simulink model "MPPT"  (R2024b)
settings: Solver=ode1  StartTime=0.0  StopTime=10  FixedStep=5e-6  RelTol=1e-3
libraries: spsSeriesRLCBranchLib x6, spsCurrentMeasurementLib x4, spsVoltageMeasurementLib x3, spsSawtoothGeneratorLib x2, spsBreakerLib x1, spsDiodeLib x1, spsGroundLib x1, spsIGBTDiodeLib x1, spsPVArrayLib x1, sps_lib x1
settings Model: Creator=DSPACE  LastModifiedBy=Ashwin Soni
settings SolverCC: AlgebraicLoopSolver=TrustRegion
settings DebuggingCC: UnconnectedInputMsg=warning  UnconnectedOutputMsg=warning  UnconnectedLineMsg=warning
settings ModelReferenceCC: EnableRefExpFcnMdlSchedulingChecks=on
settings RTWCC: GPUComputeCapability=3.5  DLArmComputeVersion=19.05

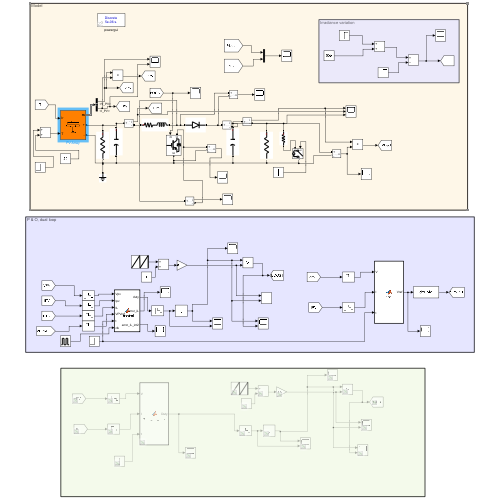
[thumbnail: Simulink's stored preview of the top-level diagram]
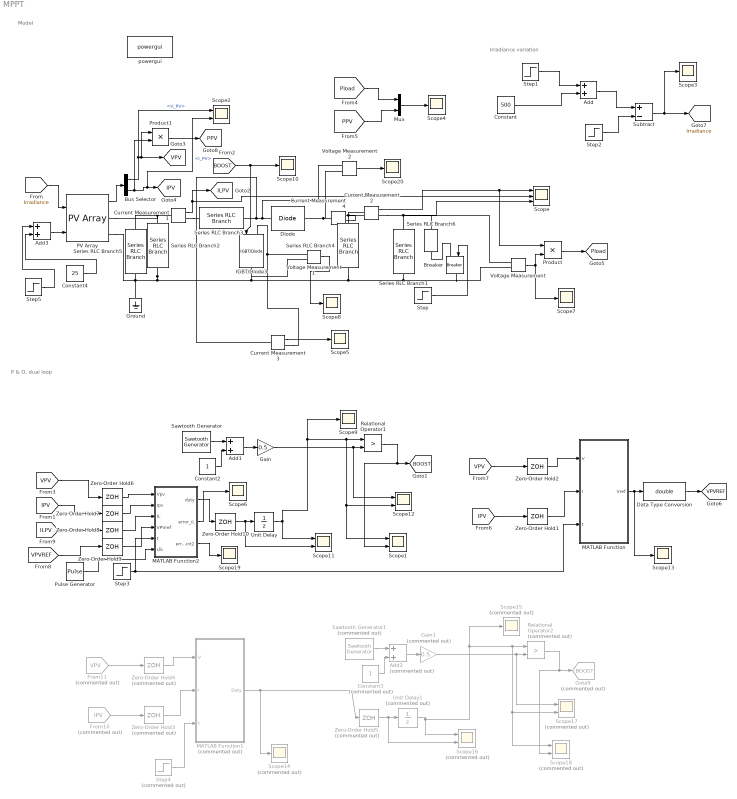
== system MPPT ==
  note: Irradiance variation
  note: Model
  note: P & O, dual loop
  Add : Sum
  Add1 : Sum
  Add2 : Sum  Commented=on
  Add3 : Sum
  Breaker : spsBreakerLib/Breaker  InitialState=0  SwitchingTimes="[1/60  5/60]"  External=on  BreakerResistance=0.01  SnubberResistance=1e6  SnubberCapacitance=inf  Measurements=None  MoreParameters=on  NoBreakLoop=off
  Bus Selector : BusSelector  OutputSignals=V_PV,I_PV
  Constant : Constant  Value=500
  Constant2 : Constant
  Constant3 : Constant  Commented=on
  Constant4 : Constant  Value=25
  Current Measurement{1..4} (4 alike) : spsCurrentMeasurementLib/Current Measurement  PhasorSimulation=off  OutputType=Complex  PSBequivalent=0
  Data Type Conversion : DataTypeConversion  OutDataTypeStr=double  SaturateOnIntegerOverflow=off  RndMeth=Floor
  Diode : spsDiodeLib/Diode  Ron=0.001  Lon=0  Vf=0.8  IC=0  UseSnubber=0  Rs=inf  Cs=250e-9  Measurements=off
  From10 : From  Commented=on  GotoTag=IPV  TagVisibility=global
  From11 : From  Commented=on  GotoTag=VPV  TagVisibility=global
  Gain : Gain  Gain=0.5
  Gain1 : Gain  Commented=on  Gain=0.5
  Goto9 : Goto  Commented=on  GotoTag=BOOST  TagVisibility=global
  Ground : spsGroundLib/Ground  LConnTagsString=a
  IGBT/Diode3 : spsIGBTDiodeLib/IGBT//Diode  Ron=75e-3  Rs=5  Cs=15e-9  Measurements=off
  MATLAB Function : MATLAB Function  TreatAsAtomicUnit=on
  MATLAB Function1 : MATLAB Function  Commented=on  TreatAsAtomicUnit=on
  MATLAB Function2 : MATLAB Function  TreatAsAtomicUnit=on
  Mux : Mux  Inputs=2
  PV Array : spsPVArrayLib/PV Array  Npar=2  Nser=2  PlotType=array @ 25 deg.C & specified irradiances  S_vec="[ 1000  800  600 ]"  Temp_C_vec="[ 45 25  ]"  ModuleName=Advance Solar Hydro Wind Power API-150  PlotWhenSelected=off  Pm=150.075  Ncell=72  Voc=41.8  Isc=5.05  Vm=34.5  Im=4.35  beta_Voc_pc=-0.419  alpha_Isc_pc=0.096  beta_Voc=-0.17514  alpha_Isc=0.004848  IL=5.0762  I0=1.155e-09  nI=1.0233  Rsh=71.9537  Rs=0.37337  RobustModel=off  RobustCellTemperature=313.3991  BAL=on  Tc=1e-6  Tfilter=5e-5
  Product : Product
  Product1 : Product
  Pulse Generator : DiscretePulseGenerator  PulseType=Time based  Period=1e-4  PulseWidth=5
  Relational Operator1 : RelationalOperator  Operator=>  OutDataTypeStr=boolean  RndMeth=Simplest  InputSameDT=off
  Relational Operator2 : RelationalOperator  Commented=on  Operator=>  OutDataTypeStr=boolean  RndMeth=Simplest  InputSameDT=off
  Sawtooth Generator : spsSawtoothGeneratorLib/Sawtooth Generator  Freq=10e3  Phase=0  Ts=0
  Sawtooth Generator1 : spsSawtoothGeneratorLib/Sawtooth Generator  Commented=on  Freq=10e3  Phase=0  Ts=0
  Scope : Scope  NumInputPorts=3
  Scope{1..2,11..12} (4 alike) : Scope  NumInputPorts=2
  Scope{3..10,13,19..20} (11 alike) : Scope
  Scope14 : Scope  Commented=on
  Scope15 : Scope  Commented=on
  Scope16 : Scope  Commented=on  NumInputPorts=2
  Scope17 : Scope  Commented=on  NumInputPorts=2
  Scope18 : Scope  Commented=on  NumInputPorts=2
  Series RLC Branch1 : spsSeriesRLCBranchLib/Series RLC Branch  LConnTagsString=__new0  RConnTagsString=__new0  BranchType=R  Resistance=100  Inductance=10e-3  SetiL0=off  InitialCurrent=0  Capacitance=1e-6  Setx0=off  InitialVoltage=0  Measurements=Branch voltage and current
  Series RLC Branch2 : spsSeriesRLCBranchLib/Series RLC Branch  LConnTagsString=__new0  RConnTagsString=__new0  BranchType=C  Resistance=1  Inductance=1e-3  SetiL0=off  InitialCurrent=0  Capacitance=220e-6  Setx0=off  InitialVoltage=0  Measurements=None
  Series RLC Branch3 : spsSeriesRLCBranchLib/Series RLC Branch  LConnTagsString=__new0  RConnTagsString=__new0  BranchType=RL  Resistance=0.05  Inductance=13.3e-3  SetiL0=off  InitialCurrent=0  Capacitance=1e-6  Setx0=off  InitialVoltage=0  Measurements=None
  Series RLC Branch4 : spsSeriesRLCBranchLib/Series RLC Branch  LConnTagsString=__new0  RConnTagsString=__new0  BranchType=C  Resistance=1  Inductance=1e-3  SetiL0=off  InitialCurrent=0  Capacitance=220e-6  Setx0=off  InitialVoltage=0  Measurements=None
  Series RLC Branch5 : spsSeriesRLCBranchLib/Series RLC Branch  LConnTagsString=__new0  RConnTagsString=__new0  BranchType=R  Resistance=10E6  Inductance=10e-3  SetiL0=off  InitialCurrent=0  Capacitance=1e-6  Setx0=off  InitialVoltage=0  Measurements=None
  Series RLC Branch6 : spsSeriesRLCBranchLib/Series RLC Branch  LConnTagsString=__new0  RConnTagsString=__new0  BranchType=R  Resistance=1000  Inductance=10e-3  SetiL0=off  InitialCurrent=0  Capacitance=1e-6  Setx0=off  InitialVoltage=0  Measurements=None
  Step : Step  Time=4  SampleTime=0
  Step1 : Step  Time=2  After=500  SampleTime=0
  Step2 : Step  Time=4  After=200  SampleTime=0
  Step3 : Step  Time=2  After=5  SampleTime=0
  Step4 : Step  Commented=on  Time=2  After=5  SampleTime=0
  Step5 : Step  Time=7  After=10  SampleTime=0
  Subtract : Sum  Inputs=+-
  Unit Delay : UnitDelay  SampleTime=1e-4  HasFrameUpgradeWarning=on
  Unit Delay1 : UnitDelay  Commented=on  SampleTime=1e-4  HasFrameUpgradeWarning=on
  Voltage Measurement : spsVoltageMeasurementLib/Voltage Measurement  PhasorSimulation=off  OutputType=Complex  PSBequivalent=0
  Voltage Measurement1 : spsVoltageMeasurementLib/Voltage Measurement  PhasorSimulation=off  OutputType=Complex  PSBequivalent=0
  Voltage Measurement2 : spsVoltageMeasurementLib/Voltage Measurement  PhasorSimulation=off  OutputType=Complex  PSBequivalent=0
  Zero-Order Hold1 : ZeroOrderHold  SampleTime=1e-2
  Zero-Order Hold{6..10} (5 alike) : ZeroOrderHold  SampleTime=1e-4
  Zero-Order Hold2 : ZeroOrderHold  SampleTime=1e-2
  Zero-Order Hold3 : ZeroOrderHold  Commented=on  SampleTime=1e-4
  Zero-Order Hold4 : ZeroOrderHold  Commented=on  SampleTime=1e-4
  Zero-Order Hold5 : ZeroOrderHold  Commented=on  SampleTime=1e-4
  powergui : sps_lib/powergui  Priority=1  SimulationMode=Discrete  SampleTime=5e-6  frequency=60  Iterations=50  frequencyindice=0  Pbase=100e6  ErrMax=1e-4  UnitsV=kV  UnitsW=MW  buscounter=0  FunctionMessages=off  echomessages=off  EnableUseOfTLC=off  CurrentSourceSwitches=off  DisableSnubberDevices=off  DisableRonSwitches=off  DisableVfSwitches=off  DisplayEquations=off  AutomaticDiscreteSolvers=off  SolverType=Tustin/Backward Euler (TBE)  Interpol=off  ExternalGateDelay=off  methode=off  Ts=100  x0status=blocks  SPID=on  SwTol=0  HookPort=off  NonlinearTolerance=1e-4  nMaxIteration=100  ContinueOnMaxIteration=off  RestoreLinks=warning  ResistiveCurrentMeasurement=off  Frange=[0:2:500]  Ylog=off  Xlog=on  ShowGrid=off  save=off  variable=ZData  structure=0  ZoomFFT=off  StartTime=0.0  cycles=1  DisplayStyle=1  fundamental=60  FreqAxis=off  MaxFrequency=1000  frequencyindicesteady=1  RmsSteady=1  display=off
  tag scope: BOOST=global, ILPV=global, IPV=global, Irradiance=global, PPV=global, Pload=global, VPV=global, VPVREF=global
  wires:
  Bus Selector/2 -> Product1/2, Scope2/2, [IPV]  "<I_PV>"
  Current Measurement1/1 -> Scope/2, [ILPV]
  PV Array/1 -> Bus Selector/1
  Bus Selector/1 -> Scope2/1, Product1/1, [VPV]  "<V_PV>"
  Current Measurement2/1 -> Product/1, Scope/1
  Gain/1 -> Scope12/1, Relational Operator1/2
  [Pload] -> Mux/1
  [VPV] -> Zero-Order Hold2/1
  [IPV] -> Zero-Order Hold1/1
  Data Type Conversion/1 -> [VPVREF]
  [IPV] -> Zero-Order Hold7/1
  [VPV] -> Zero-Order Hold6/1
  [VPVREF] -> Zero-Order Hold9/1
  [ILPV] -> Zero-Order Hold8/1
  Zero-Order Hold2/1 -> MATLAB Function/1(V)
  Zero-Order Hold1/1 -> MATLAB Function/2(I)
  [Irradiance] -> PV Array/1
  Mux/1 -> Scope4/1
  Step/1 -> Breaker/1
  Voltage Measurement/1 -> Scope7/1, Product/2
  Product/1 -> [Pload]
  Step1/1 -> Add/1
  Constant/1 -> Add/2
  Step2/1 -> Subtract/2
  Subtract/1 -> Scope3/1, [Irradiance]
  Add/1 -> Subtract/1
  [PPV] -> Mux/2
  Current Measurement3/1 -> Scope5/1
  Relational Operator1/1 -> [BOOST], Scope1/2
  Voltage Measurement1/1 -> Scope8/1
  [BOOST] -> Scope10/1, IGBT/Diode3/1
  Product1/1 -> [PPV]
  Unit Delay/1 -> Scope11/1, Scope1/1, Scope12/2, Relational Operator1/1, Scope9/1
  Zero-Order Hold6/1 -> MATLAB Function2/1(Vpv)
  Zero-Order Hold7/1 -> MATLAB Function2/2(Ipv)
  Zero-Order Hold8/1 -> MATLAB Function2/3(IL)
  Zero-Order Hold9/1 -> MATLAB Function2/4(VPVref)
  Zero-Order Hold10/1 -> Scope11/2, Unit Delay/1
  Sawtooth Generator/1 -> Add1/1
  Constant2/1 -> Add1/2
  Add1/1 -> Gain/1
  Step3/1 -> MATLAB Function/3(t), MATLAB Function2/5(t)
  MATLAB Function2/2(error_iL) -> Scope6/1
  MATLAB Function/1(Vref) -> Scope13/1, Data Type Conversion/1
  MATLAB Function2/1(duty) -> Zero-Order Hold10/1
  Zero-Order Hold4/1 -> MATLAB Function1/1(V)
  From10/1 -> Zero-Order Hold3/1
  Zero-Order Hold3/1 -> MATLAB Function1/2(I)
  MATLAB Function1/1(Duty) -> Scope14/1, Zero-Order Hold5/1
  From11/1 -> Zero-Order Hold4/1
  Add2/1 -> Gain1/1
  Unit Delay1/1 -> Scope18/1, Scope17/2, Relational Operator2/1, Scope15/1, Scope16/1
  Constant3/1 -> Add2/2
  Gain1/1 -> Scope17/1, Relational Operator2/2
  Sawtooth Generator1/1 -> Add2/1
  Relational Operator2/1 -> Scope18/2, Goto9/1
  Zero-Order Hold5/1 -> Scope16/2, Unit Delay1/1
  Step4/1 -> MATLAB Function1/3(t)
  MATLAB Function2/3(error_iL_int2) -> Scope19/1
  Pulse Generator/1 -> MATLAB Function2/6(clk)
  Constant4/1 -> Add3/2
  Step5/1 -> Add3/1
  Add3/1 -> PV Array/2
  Current Measurement4/1 -> Scope/3
  Voltage Measurement2/1 -> Scope20/1
  connections:
  Series RLC Branch2/RConn1 -- PV Array/RConn2 -- Ground/LConn1 -- Series RLC Branch5/RConn1 -- Voltage Measurement1/LConn2 -- IGBT/Diode3/RConn1 -- Breaker/RConn1 -- Voltage Measurement/LConn2 -- Series RLC Branch1/RConn1 -- Series RLC Branch4/RConn1
  Diode/LConn1 -- Voltage Measurement2/LConn1 -- Current Measurement3/LConn1 -- Series RLC Branch3/RConn1
  Series RLC Branch2/LConn1 -- PV Array/RConn1 -- Series RLC Branch5/LConn1 -- Current Measurement1/LConn1
  Current Measurement1/RConn1 -- Series RLC Branch3/LConn1
  Current Measurement2/LConn1 -- Current Measurement4/RConn1 -- Series RLC Branch4/LConn1
  Current Measurement2/RConn1 -- Series RLC Branch6/LConn1 -- Voltage Measurement/LConn1 -- Series RLC Branch1/LConn1
  Breaker/LConn1 -- Series RLC Branch6/RConn1
  Current Measurement3/RConn1 -- IGBT/Diode3/LConn1 -- Voltage Measurement1/LConn1
  Current Measurement4/LConn1 -- Diode/RConn1 -- Voltage Measurement2/LConn2

== matlab function MPPT/MATLAB Function1 ==
  data: V input; Duty output; I input; t input
% function Duty = mppt_po_duty(V, I, t)
% function Duty = mppt_po_duty(V,I,t)
% % Simple Perturb & Observe (direct duty) for BOOST converter
% % Uses only dV and dP, no filtering/MA. Tune deltaD for your plant.
% %
% % Note (BOOST): decreasing Duty -> increases Vpv, increasing Duty -> decreases Vpv.
% 
% persistent Vold Pold Dold count Vavg Pavg Iavg Vpv Ipv Ppv
% 
% % initialize persistent on first call
% if isempty(Vold)
%     Vold = V;
%     Pold = V * I;
%     Dold = 0.5;    % initial duty (70%)
%     count = 0;
%     Vpv = 0;
%     Ipv = 0;
%     Ppv = 0;
% end
% 
% % ---------- USER TUNES ----------
% deltaD = 0.005;    % step size (try 1e-4 .. 5e-4)
% Dmin   = 0.05;
% Dmax   = 0.95;
% Navg = 200;
% % ------------------------------
% 
% Vpv = Vpv + V;
% Ppv = Ppv + (V*I);
% Ipv = Ipv + I;
% 
% if(count >= Navg)
%     count = 0;
%     Vpv = Vpv/Navg;
%     Ipv = Ipv/Navg;
%     Ppv = Ppv/Navg;
% 
% % instantaneous power and deltas
% dV = Vpv - Vold;
% dP = Ppv - Pold;
% 
% % Core P&O decision (boost-sign corrected)
% if dP > 0
%     if dV > 0
%         % V increased and P increased  -> continue increasing V
%         % For boost: to increase Vpv, DECREASE duty
%         Duty = Dold - deltaD;
%     else
%         % V decreased and P increased -> continue decreasing V
%         % For boost: to decrease Vpv, INCREASE duty
%         Duty = Dold + deltaD;
%     end
% elseif dP < 0
%     if dV > 0
%         % V increased and P decreased -> reverse (decrease V)
%         Duty = Dold + deltaD;
%     else
%         % V decreased and P decreased -> reverse (increase V)
%         Duty = Dold - deltaD;
%     end
% else
%     % dP == 0 -> hold (could be MPP or flat region)
%     Duty = Dold;
% end
% 
% % apply hard bounds
% if Duty > Dmax
%     Duty = Dmax;
% elseif Duty < Dmin
%     Duty = Dmin;
% end
% 
% % update stored values
% Vold = Vpv;
% Pold = Ppv;
% Dold = Duty;
% Vpv = 0;
% Ipv = 0;
% Ppv = 0;
% 
% else
% Duty = Dold;
% count = count + 1;
% end
% 
% end
% 



function Duty = mppt_po_duty(V,I,t)
% Variable step-size Perturb & Observe MPPT for BOOST
% Uses dV and dP, adjusts deltaD: large far from MPP, small near MPP.

persistent Vold Pold Dold count Vpv Ipv Ppv

% initialize persistent on first call
if isempty(Vold)
    Vold = V;
    Pold = V * I;
    Dold = 0.5;    % initial duty
    count = 0;
    Vpv = 0; Ipv = 0; Ppv = 0;
end

% ---------- USER TUNES ----------
deltaD_max = 0.05;   % large step (far from MPP)
deltaD_min = 0.001;  % small step (near MPP)
Dmin   = 0.05;
Dmax   = 0.95;
Navg   = 500;        % averaging window
% -------------------------------

% accumulate samples
Vpv = Vpv + V;
Ppv = Ppv + (V*I);
Ipv = Ipv + I;

if(count >= Navg)
    count = 0;
    Vpv = Vpv/Navg;
    Ipv = Ipv/Navg;
    Ppv = Ppv/Navg;

    % instantaneous power and deltas
    dV = Vpv - Vold;
    dP = Ppv - Pold;

    % -------- Variable step-size --------
    % normalize |dP| relative to power level
    relChange = abs(dP) / (Ppv + 1e-6); 
    % map to deltaD range
    deltaD = deltaD_min + (deltaD_max - deltaD_min) * min(relChange,1);
    % ------------------------------------

    % Core P&O decision (boost-sign corrected)
    if dP > 0
        if dV > 0
            Duty = Dold - deltaD;  % inc V → dec duty
        else
            Duty = Dold + deltaD;  % dec V → inc duty
        end
    elseif dP < 0
        if dV > 0
            Duty = Dold + deltaD;
        else
            Duty = Dold - deltaD;
        end
    else
        Duty = Dold;
    end

    % apply bounds
    Duty = max(min(Duty, Dmax), Dmin);

    % update
    Vold = Vpv;
    Pold = Ppv;
    Dold = Duty;
    Vpv = 0; Ipv = 0; Ppv = 0;

else
    Duty = Dold;
    count = count + 1;
end
end




% function Duty = mppt_po_duty(V,I,t)
% % Hybrid Variable step-size Perturb & Observe + Incremental Conductance
% % for BOOST converter MPPT
% %
% % - Uses averaging (Navg) for stability
% % - Variable step size (deltaD shrinks near MPP)
% % - Switches to Incremental Conductance when near MPP to reduce oscillations
% 
% persistent Vold Pold Dold count Vpv Ipv Ppv Iold
% 
% % initialize persistent on first call
% if isempty(Vold)
%     Vold = V;
%     Pold = V * I;
%     Iold = I;
%     Dold = 0.5;    % initial duty
%     count = 0;
%     Vpv = 0; Ipv = 0; Ppv = 0;
% end
% 
% % ---------- USER TUNES ----------
% deltaD_max = 0.05;   % large step (far from MPP)
% deltaD_min = 0.005;  % small step (near MPP)
% Dmin   = 0.05;
% Dmax   = 0.95;
% Navg   = 500;        % averaging window
% deadbandP = 0.002;   % 0.2% power tolerance for MPP check
% deadbandSlope = 0.7; % tolerance for IncCond slope check
% % -------------------------------
% 
% % accumulate samples
% Vpv = Vpv + V;
% Ppv = Ppv + (V*I);
% Ipv = Ipv + I;
% 
% if(count >= Navg)
%     count = 0;
%     Vpv = Vpv/Navg;
%     Ipv = Ipv/Navg;
%     Ppv = Ppv/Navg;
% 
%     % instantaneous deltas
%     dV = Vpv - Vold;
%     dI = Ipv - Iold;
%     dP = Ppv - Pold;
% 
%     % -------- Variable step-size --------
%     relChange = abs(dP) / (Ppv + 1e-6); 
%     deltaD = deltaD_min + (deltaD_max - deltaD_min) * min(relChange*2,1);
%     % ------------------------------------
% 
%     % -------- Hybrid decision -----------
%     if abs(dP) < deadbandP * Ppv
%         % Near MPP -> use Incremental Conductance
%         if abs(dV) > 1e-6
%             slope = dI / dV;      % dI/dV
%             cond  = -Ipv / Vpv;   % -I/V
%             if abs(slope - cond) < deadbandSlope
%                 Duty = Dold; % At MPP, hold duty
%             elseif slope > cond
%                 Duty = Dold - deltaD; % left of MPP → dec duty (boost: inc V)
%             else
%                 Duty = Dold + deltaD; % right of MPP → inc duty (boost: dec V)
%             end
%         else
%             Duty = Dold; % no voltage change -> hold
%         end
%     else
%         % Far from MPP -> normal P&O
%         if dP > 0
%             if dV > 0
%                 Duty = Dold - deltaD;  % inc V → dec duty
%             else
%                 Duty = Dold + deltaD;  % dec V → inc duty
%             end
%         elseif dP < 0
%             if dV > 0
%                 Duty = Dold + deltaD;
%             else
%                 Duty = Dold - deltaD;
%             end
%         else
%             Duty = Dold;
%         end
%     end
%     % ------------------------------------
% 
%     % apply bounds
%     Duty = max(min(Duty, Dmax), Dmin);
% 
%     % update
%     Vold = Vpv;
%     Pold = Ppv;
%     Iold = Ipv;
%     Dold = Duty;
%     Vpv = 0; Ipv = 0; Ppv = 0;
% 
% else
%     Duty = Dold;
%     count = count + 1;
% end
% end

== matlab function MPPT/MATLAB Function ==
  data: V input; Vref output; I input; t input
function Vref = fcn(V,I,t)

Vrefmax=200;
Vrefmin=0;
Vrefinit= 69;
deltaVref=0.1;
persistent Vold Pold Vrefold;

% if(t<2)
% Vold = 0;
% Pold = 0;
% Vrefold = 0;
% Vref = 69;

% else

if isempty(Vold)
    Vold=V;
    Pold=V*I;
    Vrefold=Vrefinit;
end
P=V*I;
dV=V-Vold;
dP=P-Pold;

if dP ~= 0
    if dP>0
        if dV>0
            Vref = Vrefold + deltaVref;
        else
            Vref = Vrefold - deltaVref;
        end
    else
            if dV>0
                Vref=Vrefold - deltaVref;
            else
                Vref=Vrefold + deltaVref;
            end
     end
    
else 
    Vref = Vrefold;
end
    if Vref>=Vrefmax
        Vref=Vrefmax;
    elseif Vref <= Vrefmin
        Vref = Vrefmin;
    end
    Vrefold=Vref;
    Vold=V;
    Pold=P;
end

== matlab function MPPT/MATLAB Function2 ==
  data: Vpv input; duty output; Ipv input; IL input; VPVref input; t input; error_iL output; error_iL_int2 output; clk input
function [duty,error_iL,error_iL_int2]= picontrol(Vpv,Ipv,IL,VPVref,t,clk)

persistent error_iL_int windup IL_nmin1 IL_nmin2 duty2 error_iL2;

if(t<0)
duty = 0.0;
error_iL = 0;
error_iL_int2 = 0;
else

% gains and constants:
kp = 0.5;
ki = 20;
Ts = 1e-4; %Sampling time;
I_INT_MAX = 0.7;
I_INT_MIN = -0.7;
ILref = (Vpv*Ipv)/VPVref;

% Persistent variables for integrators

if isempty(error_iL_int)
    error_iL_int = 0;
    windup = 0;
    IL_nmin1 = 0;
    IL_nmin2 = 0;
    duty2 = 0;
    error_iL2 = 0;
end

if(clk == 1)
% control loop:
error_iL = ILref + windup - ((0.6*IL)+(0.25*IL_nmin1)+(0.15*IL_nmin2)); 
error_iL2 = error_iL;
IL_nmin2 = IL_nmin1;
IL_nmin1 = IL;
error_iL_int = error_iL_int + (error_iL*Ts); 
% if (error_iL_int > I_INT_MAX)
%             error_iL_int = I_INT_MAX;
% elseif (error_iL_int < I_INT_MIN)
%             error_iL_int = I_INT_MIN;
% end
error_iL_int2 = error_iL_int;
temp = (kp*error_iL) + (ki*error_iL_int);

if temp > 0.95
    duty = 0.95;
elseif temp < 0
    duty = 0;
else 
    duty = temp;
    duty2 = duty;
end

windup = duty - temp;


% gains and constants:

% Vpv = Vpv*100000;
% Ipv = Ipv*100000;
% IL = IL*100000;
% 
% kp = 50000;
% ki = 200000;
% Ts = 1e-4; %Sampling time;
% 
% ILref = (Vpv*Ipv)/VPVref;
% 
% % Persistent variables for integrators
% persistent error_iL_int;
% if isempty(error_iL_int)
%     error_iL_int = 0;
% end
% 
% % control loop:
% error_iL = ILref - IL; 
% error_iL_int = error_iL_int + (error_iL*Ts); 
% duty = ((kp*error_iL) + (ki*error_iL_int))/(100000*100000);
% 
% if duty > 0.95
%     duty = 0.95;
% elseif duty < 0
%     duty = 0;
% end
else
    duty = duty2;
    error_iL = error_iL2;
    error_iL_int2 = error_iL_int;
end
end
end
